simulink model "sedemo_absbrake_can"  (Simulink 7.5)
settings: Solver=ode45  SolverMode=SingleTasking  StartTime=0.0  StopTime=17  MaxStep=inf  RelTol=2e-2  AbsTol=1e-4
PreLoadFcn:
  | sedemo_absdata;
  | BUSCapacity = 50000;
StopFcn:
  | if exist ('logsout')
  | tagName = 'Net';
  | sedemo_absbrakeplots_delay;
  | clear figExt tagName;
  | end
values from neighbouring files (symbols this model uses):
  ctrl = 1    [sedemo_absdata.m]
  g = 32.18    [sedemo_absdata.m]
  I = 5    [sedemo_absdata.m]
  Kf = 1    [sedemo_absdata.m]
  m = 50    [sedemo_absdata.m]
  mu = [0 .4 .8 .97 1.0 .98 .96 .94 .92 .9 .88 .855 .83 .81 .79 .77 .75 .73 .72 .71 .7]    [sedemo_absdata.m]
  PBmax = 1500    [sedemo_absdata.m]
  Rr = 15/12    (= 1.25)    [sedemo_absdata.m]
  slip = (0:.05:1.0)    [sedemo_absdata.m]
  TB = 0.01    [sedemo_absdata.m]
  v0 = 88    [sedemo_absdata.m]
undefined symbols (not defined in the file or in its folder): des_subsystemblock, des_subsysteminport, des_subsystemoutport, des_subsystemsupportblock
libraries: simeventsrouting1 x30, simeventstranslate1 x25, simeventssink1 x21, simeventsserver1 x19, simeventsattributes2 x15, simeventsgates1 x10, simeventsqueue1 x6, simulink x5, simeventsgenerators1 x5, simeventssignalmanage1 x5, simeventstiming1 x3, simeventsinfo x1
(part 4 of 4)

== system sedemo_absbrake_can/CANbus/CAN Node 1/Flow Controller/__fcn_ss__ ==
  busy : Inport  LoadFcn=des_subsysteminport(gcb, 'load');  InitFcn=des_subsysteminport(gcb, 'init');  StartFcn=des_subsysteminport(gcb, 'start');  StopFcn=des_subsysteminport(gcb, 'stop');  OutDataType=sfix(16)  OutScaling=2^0  mask(Discrete Event Inport){PermitSubsystemEvents=on, TypeOfEvent=Sample time hit, SignalEdgeOption=Rising, SpecifyEventPriority=on, PrioritySubsystemEvent=2100}
      mask prompts: PermitSubsystemEvents "Execute subsystem upon signal-based events"; TypeOfEvent "Type of signal-based event:"; SignalEdgeOption "Type of change in signal value:"; SpecifyEventPriority "Specify event priority for executing subsystem"; PrioritySubsystemEvent "Subsystem execution event priority:"
      mask help: Input port for a Discrete Event Subsystem block. This block can conditionally execute the subsystem upon signal-based events that meet specified criteria.
      mask init:
      | des_subsystemmask(gcb, 'init','apply')
      settings: CopyFcn=des_subsysteminport(gcb, 'copy');  DeleteFcn=des_subsysteminport(gcb, 'delete');  UndoDeleteFcn=des_subsysteminport(gcb, 'undodelete');  ModelCloseFcn=des_subsysteminport(gcb, 'modelclose');  PreSaveFcn=des_subsysteminport(gcb, 'presave');  NameChangeFcn=des_subsysteminport(gcb, 'namechange');  ParentCloseFcn=des_subsysteminport(gcb, 'parentclose');
      mask Help: helpview(simeventsbhelp);
      mask StyleString: checkbox,popup(Change in signal|Trigger|Sample time hit),popup(Rising|Falling|Either),checkbox,edit
      mask CallbackString: des_subsystemmask(gcb, 'cbPermitSubsystemEvents', 'noapply');|des_subsystemmask(gcb,'cbTypeOfEvent','noapply');||des_subsystemmask(gcb, 'cbSpecifyEventPriority', 'noapply');|
  Subsystem Configuration : TriggerPort  TriggerType=function-call
      settings: CopyFcn=des_subsystemconfigblock(gcb, 'copy');  DeleteFcn=des_subsystemconfigblock(gcb, 'delete');  UndoDeleteFcn=des_subsystemconfigblock(gcb, 'undodelete');
      mask Type: Subsystem Configuration
      mask Description: Configuration for a Discrete Event Subsystem block. Every discrete event subsystem window must contain exactly one copy of this configuration block. Do not delete this block.
      mask Help: helpview(simeventsbhelp);
      mask Display: disp('Do Not Delete');
  Constant : Constant  OutDataType=sfix(16)  OutScaling=2^0
  Sum : Sum  Inputs=|-+  OutDataType=sfix(16)  OutScaling=2^0
  en : Outport  LoadFcn=des_subsystemoutport(gcb, 'load');  InitFcn=des_subsystemoutport(gcb, 'init');  StartFcn=des_subsystemoutport(gcb, 'start');  StopFcn=des_subsystemoutport(gcb, 'stop');  OutDataType=sfix(16)  OutScaling=2^0
      settings: CopyFcn=des_subsystemoutport(gcb, 'copy');  DeleteFcn=des_subsystemoutport(gcb, 'delete');  UndoDeleteFcn=des_subsystemoutport(gcb, 'undodelete');  ModelCloseFcn=des_subsystemoutport(gcb, 'modelclose');  PreSaveFcn=des_subsystemoutport(gcb, 'presave');  NameChangeFcn=des_subsystemoutport(gcb, 'namechange');  ParentCloseFcn=des_subsystemoutport(gcb, 'parentclose');
      mask Type: Discrete Event Outport
      mask Description: Provide an output port for a Discrete Event Subsystem block.
      mask Help: helpview(simeventsbhelp);
  wires:
  Sum/1 -> en/1
  Constant/1 -> Sum/2
  busy/1 -> Sum/1

== system sedemo_absbrake_can/CANbus/CAN Node 2/Error Detection/AAA___ ==

== system sedemo_absbrake_can/CANbus/CAN Node 2/Error Detection/__fcn_ss__ ==
  Rx_ID : Inport  LoadFcn=des_subsysteminport(gcb, 'load');  InitFcn=des_subsysteminport(gcb, 'init');  StartFcn=des_subsysteminport(gcb, 'start');  StopFcn=des_subsysteminport(gcb, 'stop');  OutDataType=sfix(16)  OutScaling=2^0  mask(Discrete Event Inport){PermitSubsystemEvents=off, TypeOfEvent=Sample time hit, SignalEdgeOption=Rising, SpecifyEventPriority=off, PrioritySubsystemEvent=20}
      mask prompts: PermitSubsystemEvents "Execute subsystem upon signal-based events"; TypeOfEvent "Type of signal-based event:"; SignalEdgeOption "Type of change in signal value:"; SpecifyEventPriority "Specify event priority for executing subsystem"; PrioritySubsystemEvent "Subsystem execution event priority:"
      mask help: Input port for a Discrete Event Subsystem block. This block can conditionally execute the subsystem upon signal-based events that meet specified criteria.
      mask init:
      | des_subsystemmask(gcb, 'init','apply')
      settings: CopyFcn=des_subsysteminport(gcb, 'copy');  DeleteFcn=des_subsysteminport(gcb, 'delete');  UndoDeleteFcn=des_subsysteminport(gcb, 'undodelete');  ModelCloseFcn=des_subsysteminport(gcb, 'modelclose');  PreSaveFcn=des_subsysteminport(gcb, 'presave');  NameChangeFcn=des_subsysteminport(gcb, 'namechange');  ParentCloseFcn=des_subsysteminport(gcb, 'parentclose');
      mask Help: helpview(simeventsbhelp);
      mask StyleString: checkbox,popup(Change in signal|Trigger|Sample time hit),popup(Rising|Falling|Either),checkbox,edit
      mask CallbackString: des_subsystemmask(gcb, 'cbPermitSubsystemEvents', 'noapply');|des_subsystemmask(gcb,'cbTypeOfEvent','noapply');||des_subsystemmask(gcb, 'cbSpecifyEventPriority', 'noapply');|
  Loss : Inport  LoadFcn=des_subsysteminport(gcb, 'load');  InitFcn=des_subsysteminport(gcb, 'init');  StartFcn=des_subsysteminport(gcb, 'start');  StopFcn=des_subsysteminport(gcb, 'stop');  Port=2  OutDataType=sfix(16)  OutScaling=2^0  mask(Discrete Event Inport){PermitSubsystemEvents=off, TypeOfEvent=Sample time hit, SignalEdgeOption=Rising, SpecifyEventPriority=off, PrioritySubsystemEvent=20}
      mask prompts: PermitSubsystemEvents "Execute subsystem upon signal-based events"; TypeOfEvent "Type of signal-based event:"; SignalEdgeOption "Type of change in signal value:"; SpecifyEventPriority "Specify event priority for executing subsystem"; PrioritySubsystemEvent "Subsystem execution event priority:"
      mask help: Input port for a Discrete Event Subsystem block. This block can conditionally execute the subsystem upon signal-based events that meet specified criteria.
      mask init:
      | des_subsystemmask(gcb, 'init','apply')
      settings: CopyFcn=des_subsysteminport(gcb, 'copy');  DeleteFcn=des_subsysteminport(gcb, 'delete');  UndoDeleteFcn=des_subsysteminport(gcb, 'undodelete');  ModelCloseFcn=des_subsysteminport(gcb, 'modelclose');  PreSaveFcn=des_subsysteminport(gcb, 'presave');  NameChangeFcn=des_subsysteminport(gcb, 'namechange');  ParentCloseFcn=des_subsysteminport(gcb, 'parentclose');
      mask Help: helpview(simeventsbhelp);
      mask StyleString: checkbox,popup(Change in signal|Trigger|Sample time hit),popup(Rising|Falling|Either),checkbox,edit
      mask CallbackString: des_subsystemmask(gcb, 'cbPermitSubsystemEvents', 'noapply');|des_subsystemmask(gcb,'cbTypeOfEvent','noapply');||des_subsystemmask(gcb, 'cbSpecifyEventPriority', 'noapply');|
  Rx_RTR : Inport  LoadFcn=des_subsysteminport(gcb, 'load');  InitFcn=des_subsysteminport(gcb, 'init');  StartFcn=des_subsysteminport(gcb, 'start');  StopFcn=des_subsysteminport(gcb, 'stop');  Port=3  OutDataType=sfix(16)  OutScaling=2^0  mask(Discrete Event Inport){PermitSubsystemEvents=off, TypeOfEvent=Sample time hit, SignalEdgeOption=Rising, SpecifyEventPriority=off, PrioritySubsystemEvent=20}
      mask prompts: PermitSubsystemEvents "Execute subsystem upon signal-based events"; TypeOfEvent "Type of signal-based event:"; SignalEdgeOption "Type of change in signal value:"; SpecifyEventPriority "Specify event priority for executing subsystem"; PrioritySubsystemEvent "Subsystem execution event priority:"
      mask help: Input port for a Discrete Event Subsystem block. This block can conditionally execute the subsystem upon signal-based events that meet specified criteria.
      mask init:
      | des_subsystemmask(gcb, 'init','apply')
      settings: CopyFcn=des_subsysteminport(gcb, 'copy');  DeleteFcn=des_subsysteminport(gcb, 'delete');  UndoDeleteFcn=des_subsysteminport(gcb, 'undodelete');  ModelCloseFcn=des_subsysteminport(gcb, 'modelclose');  PreSaveFcn=des_subsysteminport(gcb, 'presave');  NameChangeFcn=des_subsysteminport(gcb, 'namechange');  ParentCloseFcn=des_subsysteminport(gcb, 'parentclose');
      mask Help: helpview(simeventsbhelp);
      mask StyleString: checkbox,popup(Change in signal|Trigger|Sample time hit),popup(Rising|Falling|Either),checkbox,edit
      mask CallbackString: des_subsystemmask(gcb, 'cbPermitSubsystemEvents', 'noapply');|des_subsystemmask(gcb,'cbTypeOfEvent','noapply');||des_subsystemmask(gcb, 'cbSpecifyEventPriority', 'noapply');|
  Rx_Data : Inport  LoadFcn=des_subsysteminport(gcb, 'load');  InitFcn=des_subsysteminport(gcb, 'init');  StartFcn=des_subsysteminport(gcb, 'start');  StopFcn=des_subsysteminport(gcb, 'stop');  Port=4  OutDataType=sfix(16)  OutScaling=2^0  mask(Discrete Event Inport){PermitSubsystemEvents=on, TypeOfEvent=Sample time hit, SignalEdgeOption=Rising, SpecifyEventPriority=off, PrioritySubsystemEvent=20}
      mask prompts: PermitSubsystemEvents "Execute subsystem upon signal-based events"; TypeOfEvent "Type of signal-based event:"; SignalEdgeOption "Type of change in signal value:"; SpecifyEventPriority "Specify event priority for executing subsystem"; PrioritySubsystemEvent "Subsystem execution event priority:"
      mask help: Input port for a Discrete Event Subsystem block. This block can conditionally execute the subsystem upon signal-based events that meet specified criteria.
      mask init:
      | des_subsystemmask(gcb, 'init','apply')
      settings: CopyFcn=des_subsysteminport(gcb, 'copy');  DeleteFcn=des_subsysteminport(gcb, 'delete');  UndoDeleteFcn=des_subsysteminport(gcb, 'undodelete');  ModelCloseFcn=des_subsysteminport(gcb, 'modelclose');  PreSaveFcn=des_subsysteminport(gcb, 'presave');  NameChangeFcn=des_subsysteminport(gcb, 'namechange');  ParentCloseFcn=des_subsysteminport(gcb, 'parentclose');
      mask Help: helpview(simeventsbhelp);
      mask StyleString: checkbox,popup(Change in signal|Trigger|Sample time hit),popup(Rising|Falling|Either),checkbox,edit
      mask CallbackString: des_subsystemmask(gcb, 'cbPermitSubsystemEvents', 'noapply');|des_subsystemmask(gcb,'cbTypeOfEvent','noapply');||des_subsystemmask(gcb, 'cbSpecifyEventPriority', 'noapply');|
  Tx_ID : Inport  LoadFcn=des_subsysteminport(gcb, 'load');  InitFcn=des_subsysteminport(gcb, 'init');  StartFcn=des_subsysteminport(gcb, 'start');  StopFcn=des_subsysteminport(gcb, 'stop');  Port=5  OutDataType=sfix(16)  OutScaling=2^0  mask(Discrete Event Inport){PermitSubsystemEvents=off, TypeOfEvent=Sample time hit, SignalEdgeOption=Rising, SpecifyEventPriority=off, PrioritySubsystemEvent=20}
      mask prompts: PermitSubsystemEvents "Execute subsystem upon signal-based events"; TypeOfEvent "Type of signal-based event:"; SignalEdgeOption "Type of change in signal value:"; SpecifyEventPriority "Specify event priority for executing subsystem"; PrioritySubsystemEvent "Subsystem execution event priority:"
      mask help: Input port for a Discrete Event Subsystem block. This block can conditionally execute the subsystem upon signal-based events that meet specified criteria.
      mask init:
      | des_subsystemmask(gcb, 'init','apply')
      settings: CopyFcn=des_subsysteminport(gcb, 'copy');  DeleteFcn=des_subsysteminport(gcb, 'delete');  UndoDeleteFcn=des_subsysteminport(gcb, 'undodelete');  ModelCloseFcn=des_subsysteminport(gcb, 'modelclose');  PreSaveFcn=des_subsysteminport(gcb, 'presave');  NameChangeFcn=des_subsysteminport(gcb, 'namechange');  ParentCloseFcn=des_subsysteminport(gcb, 'parentclose');
      mask Help: helpview(simeventsbhelp);
      mask StyleString: checkbox,popup(Change in signal|Trigger|Sample time hit),popup(Rising|Falling|Either),checkbox,edit
      mask CallbackString: des_subsystemmask(gcb, 'cbPermitSubsystemEvents', 'noapply');|des_subsystemmask(gcb,'cbTypeOfEvent','noapply');||des_subsystemmask(gcb, 'cbSpecifyEventPriority', 'noapply');|
  Tx_RTR : Inport  LoadFcn=des_subsysteminport(gcb, 'load');  InitFcn=des_subsysteminport(gcb, 'init');  StartFcn=des_subsysteminport(gcb, 'start');  StopFcn=des_subsysteminport(gcb, 'stop');  Port=6  OutDataType=sfix(16)  OutScaling=2^0  mask(Discrete Event Inport){PermitSubsystemEvents=off, TypeOfEvent=Sample time hit, SignalEdgeOption=Rising, SpecifyEventPriority=off, PrioritySubsystemEvent=20}
      mask prompts: PermitSubsystemEvents "Execute subsystem upon signal-based events"; TypeOfEvent "Type of signal-based event:"; SignalEdgeOption "Type of change in signal value:"; SpecifyEventPriority "Specify event priority for executing subsystem"; PrioritySubsystemEvent "Subsystem execution event priority:"
      mask help: Input port for a Discrete Event Subsystem block. This block can conditionally execute the subsystem upon signal-based events that meet specified criteria.
      mask init:
      | des_subsystemmask(gcb, 'init','apply')
      settings: CopyFcn=des_subsysteminport(gcb, 'copy');  DeleteFcn=des_subsysteminport(gcb, 'delete');  UndoDeleteFcn=des_subsysteminport(gcb, 'undodelete');  ModelCloseFcn=des_subsysteminport(gcb, 'modelclose');  PreSaveFcn=des_subsysteminport(gcb, 'presave');  NameChangeFcn=des_subsysteminport(gcb, 'namechange');  ParentCloseFcn=des_subsysteminport(gcb, 'parentclose');
      mask Help: helpview(simeventsbhelp);
      mask StyleString: checkbox,popup(Change in signal|Trigger|Sample time hit),popup(Rising|Falling|Either),checkbox,edit
      mask CallbackString: des_subsystemmask(gcb, 'cbPermitSubsystemEvents', 'noapply');|des_subsystemmask(gcb,'cbTypeOfEvent','noapply');||des_subsystemmask(gcb, 'cbSpecifyEventPriority', 'noapply');|
  Tx_Data : Inport  LoadFcn=des_subsysteminport(gcb, 'load');  InitFcn=des_subsysteminport(gcb, 'init');  StartFcn=des_subsysteminport(gcb, 'start');  StopFcn=des_subsysteminport(gcb, 'stop');  Port=7  OutDataType=sfix(16)  OutScaling=2^0  mask(Discrete Event Inport){PermitSubsystemEvents=off, TypeOfEvent=Sample time hit, SignalEdgeOption=Rising, SpecifyEventPriority=off, PrioritySubsystemEvent=20}
      mask prompts: PermitSubsystemEvents "Execute subsystem upon signal-based events"; TypeOfEvent "Type of signal-based event:"; SignalEdgeOption "Type of change in signal value:"; SpecifyEventPriority "Specify event priority for executing subsystem"; PrioritySubsystemEvent "Subsystem execution event priority:"
      mask help: Input port for a Discrete Event Subsystem block. This block can conditionally execute the subsystem upon signal-based events that meet specified criteria.
      mask init:
      | des_subsystemmask(gcb, 'init','apply')
      settings: CopyFcn=des_subsysteminport(gcb, 'copy');  DeleteFcn=des_subsysteminport(gcb, 'delete');  UndoDeleteFcn=des_subsysteminport(gcb, 'undodelete');  ModelCloseFcn=des_subsysteminport(gcb, 'modelclose');  PreSaveFcn=des_subsysteminport(gcb, 'presave');  NameChangeFcn=des_subsysteminport(gcb, 'namechange');  ParentCloseFcn=des_subsysteminport(gcb, 'parentclose');
      mask Help: helpview(simeventsbhelp);
      mask StyleString: checkbox,popup(Change in signal|Trigger|Sample time hit),popup(Rising|Falling|Either),checkbox,edit
      mask CallbackString: des_subsystemmask(gcb, 'cbPermitSubsystemEvents', 'noapply');|des_subsystemmask(gcb,'cbTypeOfEvent','noapply');||des_subsystemmask(gcb, 'cbSpecifyEventPriority', 'noapply');|
  Subsystem Configuration : TriggerPort  TriggerType=function-call
      settings: CopyFcn=des_subsystemconfigblock(gcb, 'copy');  DeleteFcn=des_subsystemconfigblock(gcb, 'delete');  UndoDeleteFcn=des_subsystemconfigblock(gcb, 'undodelete');
      mask Type: Subsystem Configuration
      mask Description: Configuration for a Discrete Event Subsystem block. Every discrete event subsystem window must contain exactly one copy of this configuration block. Do not delete this block.
      mask Help: helpview(simeventsbhelp);
      mask Display: disp('Do Not Delete');
  Embedded MATLAB Function : Stateflow chart  TreatAsAtomicUnit=on
  Lookup Table : Lookup  InputValues=IDRange  Table=2*ones(1,length(IDRange))-IDSubscription  OutDataType=sfix(16)  OutScaling=2^0  LUTDesignUseExistingBP=off  LUTDesignAbsError=NaN
  Memory : Memory  InheritSampleTime=on
  Sum : Sum  Inputs=|++  OutDataType=sfix(16)  OutScaling=2^0
  Idx : Outport  LoadFcn=des_subsystemoutport(gcb, 'load');  InitFcn=des_subsystemoutport(gcb, 'init');  StartFcn=des_subsystemoutport(gcb, 'start');  StopFcn=des_subsystemoutport(gcb, 'stop');  OutDataType=sfix(16)  OutScaling=2^0
      settings: CopyFcn=des_subsystemoutport(gcb, 'copy');  DeleteFcn=des_subsystemoutport(gcb, 'delete');  UndoDeleteFcn=des_subsystemoutport(gcb, 'undodelete');  ModelCloseFcn=des_subsystemoutport(gcb, 'modelclose');  PreSaveFcn=des_subsystemoutport(gcb, 'presave');  NameChangeFcn=des_subsystemoutport(gcb, 'namechange');  ParentCloseFcn=des_subsystemoutport(gcb, 'parentclose');
      mask Type: Discrete Event Outport
      mask Description: Provide an output port for a Discrete Event Subsystem block.
      mask Help: helpview(simeventsbhelp);
  ACK : Outport  LoadFcn=des_subsystemoutport(gcb, 'load');  InitFcn=des_subsystemoutport(gcb, 'init');  StartFcn=des_subsystemoutport(gcb, 'start');  StopFcn=des_subsystemoutport(gcb, 'stop');  Port=2  OutDataType=sfix(16)  OutScaling=2^0
      settings: CopyFcn=des_subsystemoutport(gcb, 'copy');  DeleteFcn=des_subsystemoutport(gcb, 'delete');  UndoDeleteFcn=des_subsystemoutport(gcb, 'undodelete');  ModelCloseFcn=des_subsystemoutport(gcb, 'modelclose');  PreSaveFcn=des_subsystemoutport(gcb, 'presave');  NameChangeFcn=des_subsystemoutport(gcb, 'namechange');  ParentCloseFcn=des_subsystemoutport(gcb, 'parentclose');
      mask Type: Discrete Event Outport
      mask Description: Provide an output port for a Discrete Event Subsystem block.
      mask Help: helpview(simeventsbhelp);
  wires:
  Memory/1 -> Embedded MATLAB Function/8(Mem)
  Embedded MATLAB Function/1(ACK) -> Memory/1, ACK/1
  Tx_RTR/1 -> Embedded MATLAB Function/5(RTR1)
  Tx_Data/1 -> Embedded MATLAB Function/6(Data1)
  Tx_ID/1 -> Embedded MATLAB Function/4(ID1)
  Rx_Data/1 -> Embedded MATLAB Function/3(Data0)
  Rx_RTR/1 -> Embedded MATLAB Function/2(RTR0)
  Loss/1 -> Embedded MATLAB Function/7(Loss), Sum/2
  Lookup Table/1 -> Sum/1
  Rx_ID/1 -> Embedded MATLAB Function/1(ID0), Lookup Table/1
  Sum/1 -> Idx/1

== system sedemo_absbrake_can/CANbus/CAN Node 2/Flow Controller/AAA___ ==

== system sedemo_absbrake_can/CANbus/CAN Node 2/Flow Controller/__fcn_ss__ ==
  busy : Inport  LoadFcn=des_subsysteminport(gcb, 'load');  InitFcn=des_subsysteminport(gcb, 'init');  StartFcn=des_subsysteminport(gcb, 'start');  StopFcn=des_subsysteminport(gcb, 'stop');  OutDataType=sfix(16)  OutScaling=2^0  mask(Discrete Event Inport){PermitSubsystemEvents=on, TypeOfEvent=Sample time hit, SignalEdgeOption=Rising, SpecifyEventPriority=on, PrioritySubsystemEvent=2100}
      mask prompts: PermitSubsystemEvents "Execute subsystem upon signal-based events"; TypeOfEvent "Type of signal-based event:"; SignalEdgeOption "Type of change in signal value:"; SpecifyEventPriority "Specify event priority for executing subsystem"; PrioritySubsystemEvent "Subsystem execution event priority:"
      mask help: Input port for a Discrete Event Subsystem block. This block can conditionally execute the subsystem upon signal-based events that meet specified criteria.
      mask init:
      | des_subsystemmask(gcb, 'init','apply')
      settings: CopyFcn=des_subsysteminport(gcb, 'copy');  DeleteFcn=des_subsysteminport(gcb, 'delete');  UndoDeleteFcn=des_subsysteminport(gcb, 'undodelete');  ModelCloseFcn=des_subsysteminport(gcb, 'modelclose');  PreSaveFcn=des_subsysteminport(gcb, 'presave');  NameChangeFcn=des_subsysteminport(gcb, 'namechange');  ParentCloseFcn=des_subsysteminport(gcb, 'parentclose');
      mask Help: helpview(simeventsbhelp);
      mask StyleString: checkbox,popup(Change in signal|Trigger|Sample time hit),popup(Rising|Falling|Either),checkbox,edit
      mask CallbackString: des_subsystemmask(gcb, 'cbPermitSubsystemEvents', 'noapply');|des_subsystemmask(gcb,'cbTypeOfEvent','noapply');||des_subsystemmask(gcb, 'cbSpecifyEventPriority', 'noapply');|
  Subsystem Configuration : TriggerPort  TriggerType=function-call
      settings: CopyFcn=des_subsystemconfigblock(gcb, 'copy');  DeleteFcn=des_subsystemconfigblock(gcb, 'delete');  UndoDeleteFcn=des_subsystemconfigblock(gcb, 'undodelete');
      mask Type: Subsystem Configuration
      mask Description: Configuration for a Discrete Event Subsystem block. Every discrete event subsystem window must contain exactly one copy of this configuration block. Do not delete this block.
      mask Help: helpview(simeventsbhelp);
      mask Display: disp('Do Not Delete');
  Constant : Constant  OutDataType=sfix(16)  OutScaling=2^0
  Sum : Sum  Inputs=|-+  OutDataType=sfix(16)  OutScaling=2^0
  en : Outport  LoadFcn=des_subsystemoutport(gcb, 'load');  InitFcn=des_subsystemoutport(gcb, 'init');  StartFcn=des_subsystemoutport(gcb, 'start');  StopFcn=des_subsystemoutport(gcb, 'stop');  OutDataType=sfix(16)  OutScaling=2^0
      settings: CopyFcn=des_subsystemoutport(gcb, 'copy');  DeleteFcn=des_subsystemoutport(gcb, 'delete');  UndoDeleteFcn=des_subsystemoutport(gcb, 'undodelete');  ModelCloseFcn=des_subsystemoutport(gcb, 'modelclose');  PreSaveFcn=des_subsystemoutport(gcb, 'presave');  NameChangeFcn=des_subsystemoutport(gcb, 'namechange');  ParentCloseFcn=des_subsystemoutport(gcb, 'parentclose');
      mask Type: Discrete Event Outport
      mask Description: Provide an output port for a Discrete Event Subsystem block.
      mask Help: helpview(simeventsbhelp);
  wires:
  Sum/1 -> en/1
  Constant/1 -> Sum/2
  busy/1 -> Sum/1

== matlab function CANbus/Background Traffic/Error Detection/__fcn_ss__/Embedded MATLAB Function ==
  data: ID0 input double; ACK output double; RTR0 input double; Data0 input double; ID1 input double; RTR1 input double; Data1 input double; Loss input double; Mem input double
function ACK = fcn(ID0,RTR0,Data0,ID1,RTR1,Data1,Loss,Mem)
% This block supports an embeddable subset of the MATLAB language.
% See the help menu for details. 

% Compare the message ID, RTR, Data fields to determine whether to
% increment of decrement the ACK field.

if (ID0 == ID1 && RTR0 == RTR1 && Data0 == Data1 && Loss < 1)
    ACK = Mem + 1;
else
    ACK = Mem - 1;
end

== matlab function CANbus/CAN BUS Arbitration/Flow Controller/__fcn_ss__/Embedded MATLAB Function ==
  data: Busy input double; open output double
function open = fcn(Busy)
% This block supports an embeddable subset of the MATLAB language.
% See the help menu for details. 

open = 1 - Busy;

== matlab function CANbus/CAN Node 1/Error Detection/__fcn_ss__/Embedded MATLAB Function ==
  data: ID0 input double; ACK output double; RTR0 input double; Data0 input double; ID1 input double; RTR1 input double; Data1 input double; Loss input double; Mem input double
function ACK = fcn(ID0,RTR0,Data0,ID1,RTR1,Data1,Loss,Mem)
% This block supports an embeddable subset of the MATLAB language.
% See the help menu for details.

% Compare the message ID, RTR, Data fields to determine whether to
% increment of decrement the ACK field.

if (ID0 == ID1 && RTR0 == RTR1 && Data0 == Data1 && Loss < 1)
    ACK = Mem + 1;
else
    ACK = Mem - 1;
end

== matlab function CANbus/CAN Node 2/Error Detection/__fcn_ss__/Embedded MATLAB Function ==
  data: ID0 input double; ACK output double; RTR0 input double; Data0 input double; ID1 input double; RTR1 input double; Data1 input double; Loss input double; Mem input double
function ACK = fcn(ID0,RTR0,Data0,ID1,RTR1,Data1,Loss,Mem)
% This block supports an embeddable subset of the MATLAB language.
% See the help menu for details. 

% Compare the message ID, RTR, Data fields to determine whether to
% increment of decrement the ACK field.

if (ID0 == ID1 && RTR0 == RTR1 && Data0 == Data1 && Loss < 1)
    ACK = Mem + 1;
else
    ACK = Mem - 1;
end
